simulink model "untitled_A"  (R2013b)
settings: Solver=ode45  StartTime=0.0  StopTime=100  RelTol=1e-3
undefined symbols (not defined in the file): c, delta, Qs, R
settings Model: Creator=Yurii  LastModifiedBy=Yurii

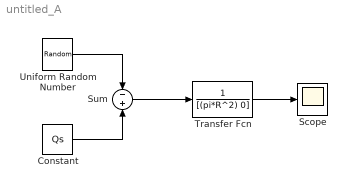
== system untitled_A ==
  Constant : Constant  Value=Qs
  Scope : Scope
  Sum : Sum  Inputs=-|+
  Transfer Fcn : TransferFcn  Denominator=[(pi*R^2) 0]
  Uniform Random Number : UniformRandomNumber  Minimum=(c-delta)*Qs  Maximum=(c+delta)*Qs  SampleTime=0.1
  wires:
  Constant/1 -> Sum/2
  Uniform Random Number/1 -> Sum/1
  Sum/1 -> Transfer Fcn/1
  Transfer Fcn/1 -> Scope/1
